simulink model "hil_node"  (Simulink 7.8)
settings: Solver=FixedStepDiscrete  SolverMode=SingleTasking  StartTime=0.0  StopTime=10.0  FixedStep=0.01  RelTol=1e-3
InitFcn:
  | clear all
  | common
undefined symbols (not defined in the file): cpInitCommunications, HilNodeInit, Init_onlyOnce, Init_Reset
libraries: dsPICdrivers x7, ecan_dspic x1, simulink x1
CloseFcn:
  | rtwprivate ssgencode ModelCloseRequest code_gen
settings Model: Creator=bwmairs  LastModifiedBy=Bryant
settings OptimizationCC: BlockReduction=off  InlineParams=on  InlineInvariantSignals=on  PassReuseOutputArgsAs=Individual arguments  ZeroExternalMemoryAtStartup=off  ZeroInternalMemoryAtStartup=off  InitFltsAndDblsToZero=on  NoFixptDivByZeroProtection=on  EfficientFloat2IntCast=on  OptimizeModelRefInitCode=on
settings DebuggingCC: ReadBeforeWriteMsg=DisableAll  WriteAfterWriteMsg=DisableAll  WriteAfterReadMsg=DisableAll  UnderspecifiedInitializationDetection=Simplified  ParameterOverflowMsg=warning  FcnCallInpInsideContextMsg=Use local settings  UniqueDataStoreMsg=error
settings HardwareCC: ProdBitPerInt=16  ProdBitPerPointer=16  ProdIntDivRoundTo=Zero  ProdEndianess=LittleEndian  ProdWordSize=16  ProdHWDeviceType=16-bit Generic
settings ModelReferenceCC: ModelReferenceNumInstancesAllowed=Single
settings SFSimCC: SimParseCustomCode=off
settings RTWCC: SystemTargetFile=dspic.tlc  GenCodeOnly=on  MakeCommand=make_CreateMPLAB  TemplateMakefile=dspic_pic30_gcc.tmf  PostCodeGenCommand=dsPIC_Compile()  Description=Embedded Target for Microchip dsPIC (real-time)  ProcessScript=dspic_make_rtw_hook  RTWCompilerOptimization=On
settings RTWCC: CustomInclude=|
  | ../../../mavlink/C/include_v1.0/sealion
  | clib
  | ../Libs/C
  | ../../../ECAN_dspic
settings RTWCC: CustomSource=|
  | clib/HilNode.c
  | clib/EcanSensors.c
  | clib/CommProtocol.c
  | 
  | ../Libs/C/Node.c
  | ../Libs/C/MessageScheduler.c
  | ../Libs/C/Conversions.c
  | ../Libs/C/Nmea2000.c
  | ../Libs/C/Nmea2000Encode.c
  | ../Libs/C/Rudder.c
  | ../Libs/C/Uart1.c
  | ../Libs/C/CanMessages.c
  | ../Libs/C/Traps.c
  | ../Libs/C/DEE.c
  | ../Libs/C/DEES.s
  | 
  | ../../../ECAN_dspic/CircularBuffer.c
  | ../../../ECAN_dspic/ecanFunctions.c
settings CodeAppCC: IgnoreCustomStorageClasses=off  IgnoreTestpoints=on
settings STFCustomTargetCC: TargetFunctionLibrary=C89/C90 (ANSI)  IncludeMdlTerminateFcn=off  GeneratePreprocessorConditionals=Use local settings  CombineOutputUpdateFcns=on  SuppressErrorStatus=on  ERTCustomFileBanners=on  SupportComplex=off  SupportContinuousTime=off  SupportNonInlinedSFcns=off  SystemTargetFile=dspic.tlc
settings ERTTargetCC: TargetFunctionLibrary=C89/C90 (ANSI)  MultiwordLength=2048  ParMdlRefBuildCompliant=off  CompOptLevelCompliant=off  ConcurrentExecutionCompliant=off  IncludeMdlTerminateFcn=off  SuppressErrorStatus=on  ERTFirstTimeCompliant=off  SupportComplex=off  ModelStepFunctionPrototypeControlCompliant=off  CPPClassGenCompliant=off  ExtModeMexFile=ext_serial_win32_comm  InlinedParameterPlacement=NonHierarchical  ERTSrcFileBannerTemplate=dsPIC_code_template.cgt  ERTHdrFileBannerTemplate=dsPIC_code_template.cgt  ERTDataSrcFileTemplate=dsPIC_code_template.cgt  ERTDataHdrFileTemplate=dsPIC_code_template.cgt  ERTCustomFileTemplate=dsPIC_main.tlc  SuppressUnreachableDefaultCases=off
settings CustomProperty: DataType=string  Value=C:\PROGRA~1\MATLAB\R2011b\bin\win64\gmake

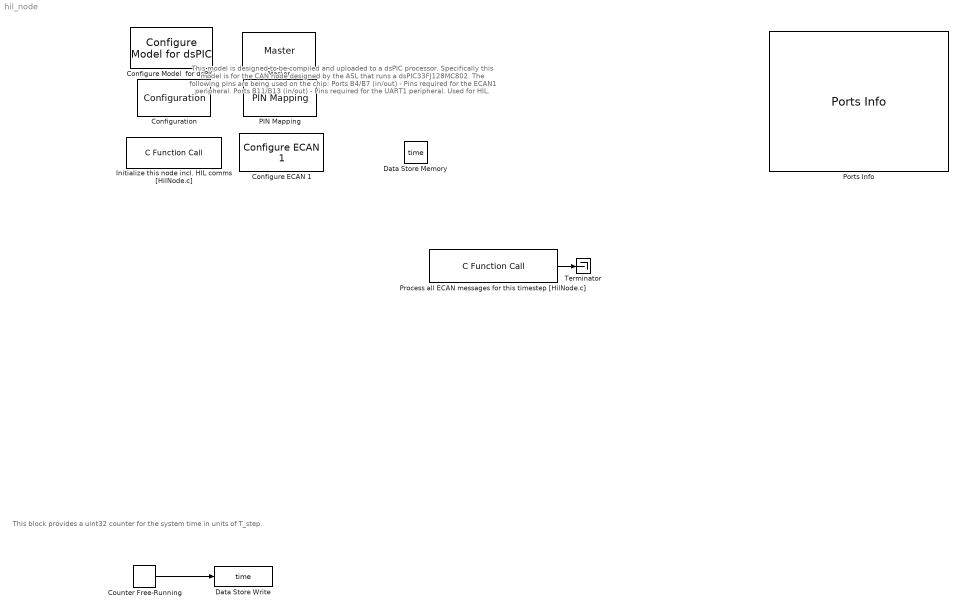
== system hil_node ==
  note: This model is designed to be compiled and uploaded to a dsPIC processor.
      | Specifically this model is for the CAN node designed by the ASL that runs a dsPIC33FJ128MC802.
      | The following pins are being used on the chip:
      | Ports B4/B7 (in/out) - Pins required for the ECAN1 peripheral.
      | Ports B11/B13 (in/out) - Pins required for the UART1 peripheral. Used for HIL.
  note: This block provides a uint32 counter for the system time in units of T_step.
  Configuration : dsPICdrivers/Configuration  double64=on
  Configure ECAN 1 : ecan_dspic/Configure ECAN 1  frame_setting=on  mode=Normal  dma_rx_chan=2  dma_tx_chan=0  baud=250000  ps1=8  pd=5  ps2=6  sjw=4  tq=20  triple_sample=on  dma_buf_size=4 buffers  rx_bufs=[1]  tx_bufs=[0]  buf_0_tx_pri=Highest  buf_0_rte=No  buf_1_tx_pri=Highest  buf_1_rte=No  buf_2_tx_pri=Lowest  buf_2_rte=No  buf_3_tx_pri=Lowest  buf_3_rte=No  buf_4_tx_pri=Lowest  buf_4_rte=No  buf_5_tx_pri=Lowest  buf_5_rte=No  buf_6_tx_pri=Lowest  buf_6_rte=No  buf_7_tx_pri=Lowest  buf_7_rte=No  mask_0=0  mask_0_mide=Match std or ext  mask_1=0  mask_1_mide=Match std or ext  mask_2=0  mask_2_mide=Match std or ext  filters=[0]  filter_0=0  filter_0_mask=0  filter_0_exide=Match only standard  filter_0_buf=1  filter_1=hex2dec('401')  filter_1_mask=0  filter_1_exide=Match only standard  filter_1_buf=2  filter_2=hex2dec('402')  filter_2_mask=0  filter_2_exide=Match only standard  filter_2_buf=3  filter_3=0  filter_3_mask=0  filter_3_exide=Match only standard  filter_3_buf=0  filter_4=0  filter_4_mask=0  filter_4_exide=Match only standard  filter_4_buf=0  filter_5=0  filter_5_mask=0  filter_5_exide=Match only standard  filter_5_buf=0  filter_6=0  filter_6_mask=0  filter_6_exide=Match only standard  filter_6_buf=0  filter_7=0  filter_7_mask=0  filter_7_exide=Match only standard  filter_7_buf=0  filter_8=0  filter_8_mask=0  filter_8_exide=Match only standard  filter_8_buf=0  filter_9=0  filter_9_mask=<empty>  filter_9_exide=Match only standard  filter_9_buf=0  filter_10=0  filter_10_mask=0  filter_10_exide=Match only standard  filter_10_buf=0  filter_11=0  filter_11_mask=0  filter_11_exide=Match only standard  filter_11_buf=0  filter_12=0  filter_12_mask=0  filter_12_exide=Match only standard  filter_12_buf=0  filter_13=0  filter_13_mask=0  filter_13_exide=Match only standard  filter_13_buf=0  filter_14=0  filter_14_mask=0  filter_14_exide=Match only standard  filter_14_buf=0  filter_15=0  filter_15_mask=0  filter_15_exide=Match only standard  filter_15_buf=0
  Configure Model  for dsPIC : dsPICdrivers/Simulink Configuration/Configure Model  for dsPIC
  Counter Free-Running : simulink/Sources/Counter Free-Running  NumBits=32  tsamp=T_step
  Data Store Memory : DataStoreMemory  DataStoreName=time  ReadBeforeWriteMsg=warning  WriteAfterWriteMsg=warning  WriteAfterReadMsg=warning  OutDataTypeStr=uint32
      settings: RTWStateStorageClass=ImportedExtern
  Data Store Write : DataStoreWrite  DataStoreName=time  DataStoreElements=time
  Initialize this node incl. HIL comms [HilNode.c] : dsPICdrivers/OTHERS/C Function Call  Tag=dsPIC_dsPIC_CFunctionCall  FctUpdate=None  fctName=cpInitCommunications  INPUT_SIZE=1  INPUT1=--  INPUT2=--  INPUT3=--  OUTPUT_SIZE=1  OUTPUT1=--  SampleTime=Inf  InputType=[]  OutputType=[]  FctDeclaration=extern void cpInitCommunications();  FctCall=cpInitCommunications();  OrderingInOutPopup=None  FctStart=Start Function (Call once and only once)  FctStart_Name=HilNodeInit  FctStart_Declaration=inline extern void HilNodeInit();  FctStart_Call=HilNodeInit();  FctInit=None  FctInit_Name=Init_Reset  FctInit_Declaration=inline extern void Init_Reset();  FctInit_Call=Init_Reset();  PinDigitalInput=[]  PinDigitalOutput=[]  AnalogueInput=[]
  Master : dsPICdrivers/Master  Tag=dsPIC_MASTER  Priority=1  TimeStepType=Timer1  picType=33fj128MC802  fcy=40008571.4286  Quartz_33f=8e6  PLLActive_33f=on  fcyDesired_33f=40000000  tmr1="[8  50010  -0.00057131]"  tmr1Info="Time Step : 0.01  ;   Error : -0.00057131%  PR1=50010"  tmr2345="[0  0  0  0]"  tmr2345cfg=[-1 -1 -1 -1]  IOautoConf=on  typePort="[ 0   0   0   0   0   0   0   0   0   0   0   0   0   0   0   0   0   0   0   0  22   0   0  23   0   0   0  23   0  22   0   0   0   0   0   0   0   0   0   0   0   0   0   0   0   0   0   0   0   0   0   0   0   0   0   0   0   0   0   0   0   0   0   0   0   0   0   0   0   0   0   0   0   0   0   0   0   0   0   0   0   0   0   0   0   0   0   0   0   0   0   0   0   0   0   0   0   0   0   0   0   0   0   0   0   0   0   0   0   0   0   0 ]"  TRIS="[ 65535  63359  65535  65535  65535  65535  65535 ]"  ADPCFG=0  MasterBusyPort=None  MasterOverloadPort=None  FOSC=Internal Fast RC 7.37Mhz  ClockSwitchMonitor=Both disabled  TempProtection_33f=TEMP_ON  FPBOR=<empty>  PWRT=disable  MCLR=<empty>  ICD=ICS_PGD3  JTAGEN=JTAGEN_OFF  PowerSave=off  OverrideFcy=off  NewFcy=1e6  PR2345="[65535  65535  65535  65535]"
  PIN Mapping : dsPICdrivers/Peripheral MAPPING/PIN Mapping  Tag=dsPIC_PIN_Mapping  in_INT1=Not tied (VSS)  in_INT2=Not tied (VSS)  in_T2CK=Not tied (VSS)  in_T3CK=Not tied (VSS)  in_T4CK=Not tied (VSS)  in_T5CK=Not tied (VSS)  in_IC1=Not tied (VSS)  in_IC2=Not tied (VSS)  in_IC7=Not tied (VSS)  in_IC8=Not tied (VSS)  out_OC1=Not changed  out_OC2=Not changed  out_OC3=Not changed  out_OC4=Not changed  in_OCFA=Not tied (VSS)  in_FLTA1=Not tied (VSS)  in_FLTA2=Not tied (VSS)  in_QEA1=Not tied (VSS)  in_QEB1=Not tied (VSS)  in_INDX1=Not tied (VSS)  out_UPDN1=Not changed  out_UPDN2=Not changed  in_QEA2=Not tied (VSS)  in_QEB2=Not tied (VSS)  in_INDX2=Not tied (VSS)  in_U1RX=tied to RP13  out_U1TX=tied to RP11  in_U1CTS=Not tied (VSS)  out_U1RTS=Not changed  in_U2RX=Not tied (VSS)  out_U2TX=Not changed  in_U2CTS=Not tied (VSS)  out_U2RTS=Not changed  in_SDI1=Not tied (VSS)  out_SDO1=Not changed  in_SCK1=Not tied (VSS)  out_SCK1OUT=Not changed  in_SS1=Not tied (VSS)  out_SS1OUT=Not changed  in_SDI2=Not tied (VSS)  out_SDO2=Not changed  in_SCK2=Not tied (VSS)  out_SCK2OUT=Not changed  in_SS2=Not tied (VSS)  out_SS2OUT=Not changed  in_C1RX=tied to RP4  out_C1TX=tied to RP7  out_C1OUT=Not changed  out_C2OUT=Not changed
  Ports Info : dsPICdrivers/Ports Info  Tag=dsPIC_PortInfo
  Process all ECAN messages for this timestep [HilNode.c] : dsPICdrivers/OTHERS/C Function Call  Tag=dsPIC_dsPIC_CFunctionCall  FctUpdate=Output Function  fctName=ProcessAllEcanMessages  INPUT_SIZE=1  INPUT1=--  INPUT2=--  INPUT3=--  OUTPUT_SIZE=1  OUTPUT1=uint8  SampleTime=.01  InputType=[ ]  OutputType=[ 2 ]  FctDeclaration=extern uint8_T ProcessAllEcanMessages();  FctCall=%y1 = ProcessAllEcanMessages();  OrderingInOutPopup=None  FctStart=None  FctStart_Name=Init_onlyOnce  FctStart_Declaration=inline extern void Init_onlyOnce();  FctStart_Call=Init_onlyOnce();  FctInit=None  FctInit_Name=Init_Reset  FctInit_Declaration=inline extern void Init_Reset();  FctInit_Call=Init_Reset();  PinDigitalInput=[]  PinDigitalOutput=[]  AnalogueInput=[]
  Terminator : Terminator
  wires:
  Counter Free-Running/1 -> Data Store Write/1
  Process all ECAN messages for this timestep [HilNode.c]/1 -> Terminator/1
